simulink model "model_rider"  (Simulink 7.4)
settings: Solver=ode23s  StartTime=0.0  StopTime=30  FixedStep=Ts  RelTol=1e-3
values from neighbouring files (symbols this model uses):
  Kdelta = 60.0000    (= 60)    [main_hess.m]    (also in main_rider.m; main_rider_time.m = 39; matlab.mat)
  Kn = 0    [main_hess.m]    (also in main_rider.m = 1; matlab.mat = 1)
  Kphi = 8.5460    (= 8.546)    [main_hess.m]    (also in main_rider.m; main_rider_time.m = 9.975; matlab.mat)
  Kphid = -0.0750    (= -0.075)    [main_hess.m]    (also in main_rider.m; main_rider_time.m = -0.07; matlab.mat)
  Kpsi = .1651    (= 0.1651)    [main_hess.m]    (also in main_rider.m; main_rider_time.m = 0.1585; matlab.mat)
  Ky = .1021    (= 0.1021)    [main_hess.m]    (also in main_rider.m; main_rider_time.m = 0.1014; matlab.mat)
  Ts = 1/Fs    [definitions.m]    (also in main_hess.m = 0.05; main_mimo.m = 0.1; main_rider.m = 0.02; main_rider_time.m = 0.02)
  v = 5    [main_hess.m]    (also in main_mimo.m; main_rider.m; main_rider_time.m; main_siso.m)
libraries: cstblocks x2, simulink x1
settings Model: Creator=Peter  LastModifiedBy=Peter
settings DataIOCC: SaveOutput=off  SaveTime=off

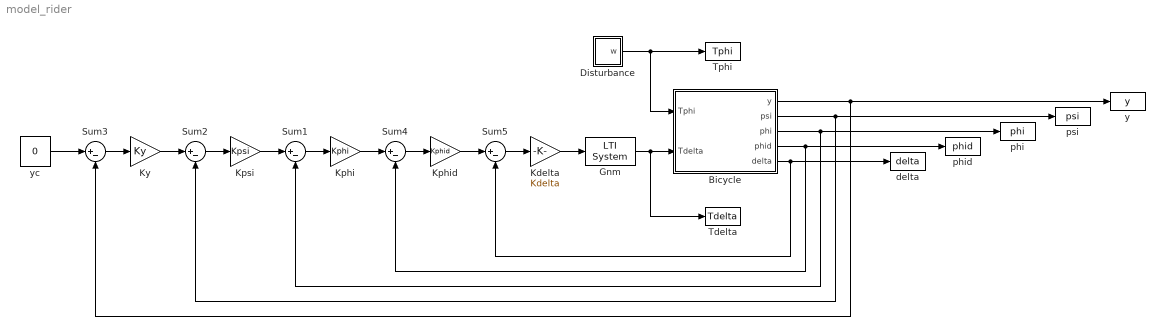
== system model_rider ==
  Bicycle : Subsystem  mask{v=v, Ts=Ts}
  Disturbance : Subsystem  mask{Ts=Ts}
  Gnm : cstblocks/LTI System  SystemSampleTime=-1  sys=Gnm  IC=[]
  Kdelta : Gain  Gain=Kdelta  ParameterDataType=fixdt(1, 16)  ParameterScaling=2^0  OutDataType=fixdt(1, 16)  OutScaling=2^0
  Kphi : Gain  Gain=Kphi  ParameterDataType=fixdt(1, 16)  ParameterScaling=2^0  OutDataType=fixdt(1, 16)  OutScaling=2^0
  Kphid : Gain  Gain=Kphid  ParameterDataType=fixdt(1, 16)  ParameterScaling=2^0  OutDataType=fixdt(1, 16)  OutScaling=2^0
  Kpsi : Gain  Gain=Kpsi  ParameterDataType=fixdt(1, 16)  ParameterScaling=2^0  OutDataType=fixdt(1, 16)  OutScaling=2^0
  Ky : Gain  Gain=Ky  ParameterDataType=fixdt(1, 16)  ParameterScaling=2^0  OutDataType=fixdt(1, 16)  OutScaling=2^0
  Sum{1..5} (5 alike) : Sum  Inputs=|+-  OutDataType=fixdt(1, 16)  OutScaling=2^0
  Tdelta : ToWorkspace  VariableName=Tdelta  SampleTime=Ts  SaveFormat=Array
  Tphi : ToWorkspace  VariableName=Tphi  SampleTime=Ts  SaveFormat=Array
  delta : ToWorkspace  VariableName=delta  SampleTime=Ts  SaveFormat=Array
  phi : ToWorkspace  VariableName=phi  SampleTime=Ts  SaveFormat=Array
  phid : ToWorkspace  VariableName=phid  SampleTime=Ts  SaveFormat=Array
  psi : ToWorkspace  VariableName=psi  SampleTime=Ts  SaveFormat=Array
  y : ToWorkspace  VariableName=y  SampleTime=Ts  SaveFormat=Array
  yc : Constant  Value=0  OutDataType=fixdt(1, 16)  OutScaling=2^0  SampleTime=Ts
  wires:
  Kpsi/1 -> Sum1/1
  Sum1/1 -> Kphi/1
  Disturbance/1(w) -> Bicycle/1(Tphi), Tphi/1
  Sum3/1 -> Ky/1
  Ky/1 -> Sum2/1
  Sum2/1 -> Kpsi/1
  yc/1 -> Sum3/1
  Sum4/1 -> Kphid/1
  Kphi/1 -> Sum4/1
  Kphid/1 -> Sum5/1
  Sum5/1 -> Kdelta/1
  Kdelta/1 -> Gnm/1
  Gnm/1 -> Bicycle/2(Tdelta), Tdelta/1
  Bicycle/5(delta) -> Sum5/2, delta/1
  Bicycle/4(phid) -> Sum4/2, phid/1
  Bicycle/3(phi) -> Sum1/2, phi/1
  Bicycle/2(psi) -> Sum2/2, psi/1
  Bicycle/1(y) -> Sum3/2, y/1

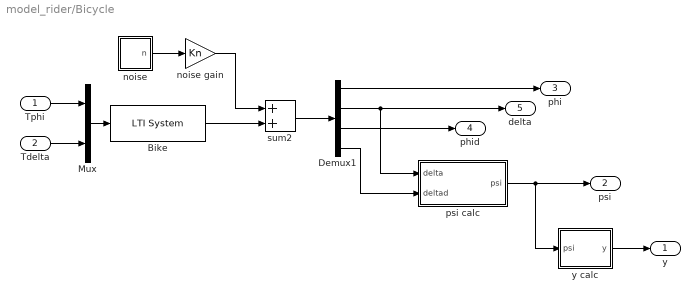
== system model_rider/Bicycle ==
  Tphi : Inport  OutDataType=fixdt(1, 16)  OutScaling=2^0
  Tdelta : Inport  Port=2  OutDataType=fixdt(1, 16)  OutScaling=2^0
  Bike : cstblocks/LTI System  SystemSampleTime=-1  sys=bike  IC=zeros(4,1);
  Demux1 : Demux
  Mux : Mux  Inputs=2
  noise : Subsystem  mask{Ts=Ts}
  noise gain : Gain  Gain=Kn  ParameterDataType=sfix(16)  ParameterScaling=2^0  OutDataType=sfix(16)  OutScaling=2^0
  psi calc : Subsystem  mask{v=v}
  sum2 : Sum  OutDataType=sfix(16)  OutScaling=2^0  SaturateOnIntegerOverflow=on  InputSameDT=on  OutDataTypeStr=Inherit: Same as first input
  y calc : Subsystem  mask{v=v}
  y : Outport  OutDataType=fixdt(1, 16)  OutScaling=2^0
  psi : Outport  Port=2  OutDataType=fixdt(1, 16)  OutScaling=2^0
  phi : Outport  Port=3  OutDataType=fixdt(1, 16)  OutScaling=2^0
  phid : Outport  Port=4  OutDataType=fixdt(1, 16)  OutScaling=2^0
  delta : Outport  Port=5  OutDataType=fixdt(1, 16)  OutScaling=2^0
  wires:
  Tphi/1 -> Mux/1
  Tdelta/1 -> Mux/2
  Mux/1 -> Bike/1
  noise/1(n) -> noise gain/1
  noise gain/1 -> sum2/1
  Bike/1 -> sum2/2
  sum2/1 -> Demux1/1
  psi calc/1(psi) -> psi/1, y calc/1(psi)
  Demux1/2 -> delta/1, psi calc/1(delta)
  Demux1/4 -> psi calc/2(deltad)
  Demux1/1 -> phi/1
  Demux1/3 -> phid/1
  y calc/1(y) -> y/1

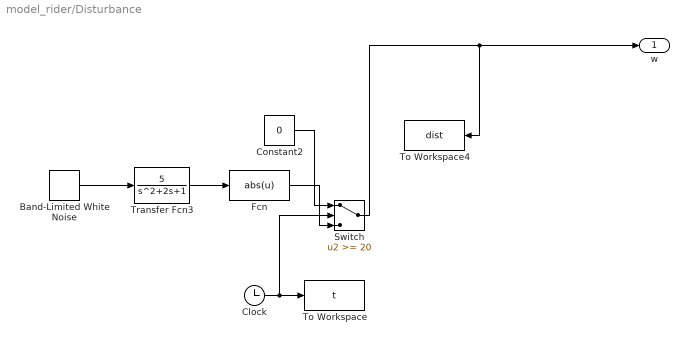
== system model_rider/Disturbance ==
  Band-Limited White Noise : simulink/Sources/Band-Limited White Noise  SystemSampleTime=-1  Cov=[0.1]  Ts=Ts  seed=[12457]
  Clock : Clock
      settings: Decimation=10
  Constant2 : Constant  Value=0  OutDataType=sfix(16)  OutScaling=2^0
  Fcn : Fcn  Expr=abs(u)
  Switch : Switch  Threshold=20
  To Workspace : ToWorkspace  VariableName=t  SampleTime=Ts  SaveFormat=Array
  To Workspace4 : ToWorkspace  VariableName=dist  SampleTime=.05  SaveFormat=Array
  Transfer Fcn3 : TransferFcn  Numerator=5
  w : Outport  OutDataType=fixdt(1, 16)  OutScaling=2^0
  wires:
  Clock/1 -> To Workspace/1, Switch/2
  Band-Limited White Noise/1 -> Transfer Fcn3/1
  Constant2/1 -> Switch/1
  Transfer Fcn3/1 -> Fcn/1
  Switch/1 -> To Workspace4/1, w/1
  Fcn/1 -> Switch/3

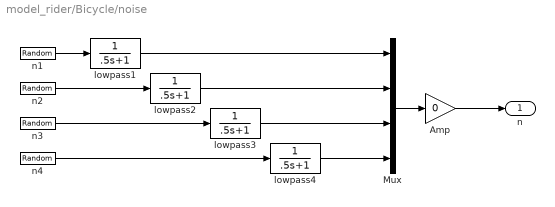
== system model_rider/Bicycle/noise ==
  Amp : Gain  Gain=0  ParameterDataType=fixdt(1, 16)  ParameterScaling=2^0  OutDataType=fixdt(1, 16)  OutScaling=2^0
  Mux : Mux
  lowpass{1..4} (4 alike) : TransferFcn  Denominator=[.5 1]
  n{1..4} (4 alike) : RandomNumber  Seed=61  SampleTime=Ts
  n : Outport  OutDataType=fixdt(1, 16)  OutScaling=2^0
  wires:
  Mux/1 -> Amp/1
  n1/1 -> lowpass1/1
  n2/1 -> lowpass2/1
  n3/1 -> lowpass3/1
  Amp/1 -> n/1
  n4/1 -> lowpass4/1
  lowpass1/1 -> Mux/1
  lowpass2/1 -> Mux/2
  lowpass3/1 -> Mux/3
  lowpass4/1 -> Mux/4

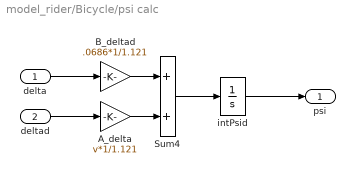
== system model_rider/Bicycle/psi calc ==
  delta : Inport  OutDataType=fixdt(1, 16)  OutScaling=2^0
  deltad : Inport  Port=2  OutDataType=fixdt(1, 16)  OutScaling=2^0
  A_delta : Gain  Gain=v*1/1.121  ParameterDataType=sfix(16)  ParameterScaling=2^0  OutDataType=sfix(16)  OutScaling=2^0
  B_deltad : Gain  Gain=.0686*1/1.121  ParameterDataType=sfix(16)  ParameterScaling=2^0  OutDataType=sfix(16)  OutScaling=2^0
  Sum4 : Sum  OutDataType=sfix(16)  OutScaling=2^0
  intPsid : TransferFcn  Numerator=1  Denominator=[1 0]
  psi : Outport  OutDataType=fixdt(1, 16)  OutScaling=2^0
  wires:
  B_deltad/1 -> Sum4/1
  A_delta/1 -> Sum4/2
  Sum4/1 -> intPsid/1
  delta/1 -> B_deltad/1
  deltad/1 -> A_delta/1
  intPsid/1 -> psi/1

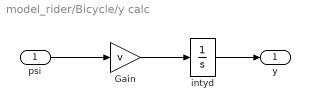
== system model_rider/Bicycle/y calc ==
  psi : Inport  OutDataType=fixdt(1, 16)  OutScaling=2^0
  Gain : Gain  Gain=v  ParameterDataType=fixdt(1, 16)  ParameterScaling=2^0  OutDataType=fixdt(1, 16)  OutScaling=2^0
  intyd : TransferFcn  Numerator=1  Denominator=[1 0]
  y : Outport  OutDataType=fixdt(1, 16)  OutScaling=2^0
  wires:
  psi/1 -> Gain/1
  Gain/1 -> intyd/1
  intyd/1 -> y/1
